simulink model "lead_phase_for_motor_system"  (R2022b)
settings: Solver=VariableStepAuto  StartTime=0.0  StopTime=10.0  RelTol=1e-3
settings Model: Creator=ZJX  LastModifiedBy=ZJX

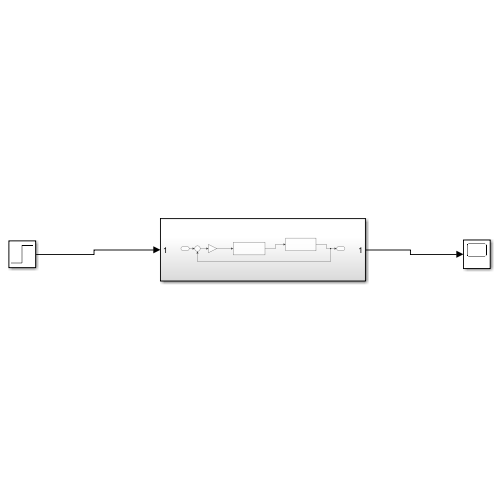
[thumbnail: Simulink's stored preview of the top-level diagram]
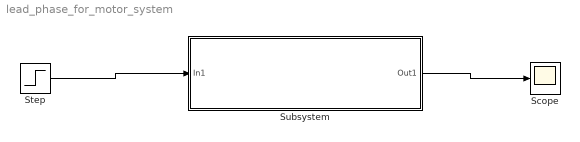
== system lead_phase_for_motor_system ==
  Scope : Scope
  Step : Step  SampleTime=0
  Subsystem : Subsystem
  wires:
  Step/1 -> Subsystem/1(In1)
  Subsystem/1(Out1) -> Scope/1

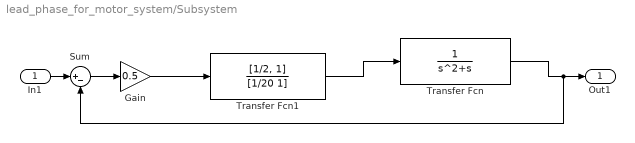
== system lead_phase_for_motor_system/Subsystem ==
  In1 : Inport
  Gain : Gain  Gain=0.5
  Sum : Sum  Inputs=|+-
  Transfer Fcn : TransferFcn  Denominator=[1 1 0]
  Transfer Fcn1 : TransferFcn  Numerator=[1/2, 1]  Denominator=[1/20 1]
  Out1 : Outport
  wires:
  Transfer Fcn/1 -> Sum/2, Out1/1
  Transfer Fcn1/1 -> Transfer Fcn/1
  Gain/1 -> Transfer Fcn1/1
  In1/1 -> Sum/1
  Sum/1 -> Gain/1
